simulink model "LUTtest"  (R2021b)
settings: Solver=FixedStepAuto  StartTime=0.0  StopTime=20  RelTol=1e-3  EnableMultiTasking=on
model workspace (MAT data in the model file):
  lutSpeed = Simulink.LookupTable
  lutSpeed.Table = Simulink.lookuptable.Table
  lutSpeed.Table.Value = [-0.999909204263 -0.999329299739 -0.995054753687 -0.964027580076 -0.761594155956 0 0.761594155956 0.964027580076 0.995054753687 0.999329299739 0.999909204263]
  lutSpeed.Table.Dimensions = [1 11]
  lutSpeed.Table.DataType = 'auto'
  lutSpeed.Table.FieldName = 'Table'
  lutSpeed.Breakpoints = Simulink.lookuptable.Breakpoint
  lutSpeed.Breakpoints.Value = [-5 -4 -3 -2 -1 0 1 2 3 4 5]
  lutSpeed.Breakpoints.TunableSizeName = 'N1'
  lutSpeed.Breakpoints.Dimensions = [1 11]
  lutSpeed.Breakpoints.DataType = 'auto'
  lutSpeed.Breakpoints.FieldName = 'BP1'
  lutSpeed.SupportTunableSize = 0
  lutSpeed.StructTypeInfo = Simulink.lookuptable.StructTypeInfo
  lutSpeed.StructTypeInfo.Name = 'lutSpeed'
  lutSpeed.StructTypeInfo.DataScope = 'Auto'
  pwm_speed = Simulink.LookupTable
  pwm_speed.Table = Simulink.lookuptable.Table
  pwm_speed.Table.Value = [-0.999909204263 -0.999329299739 -0.995054753687 -0.964027580076 -0.761594155956 0 0.761594155956 0.964027580076 0.995054753687 0.999329299739 0.999909204263]
  pwm_speed.Table.Dimensions = [1 11]
  pwm_speed.Table.DataType = 'auto'
  pwm_speed.Table.FieldName = 'Table'
  pwm_speed.Breakpoints = Simulink.lookuptable.Breakpoint
  pwm_speed.Breakpoints.Value = [-5 -4 -3 -2 -1 0 1 2 3 4 5]
  pwm_speed.Breakpoints.TunableSizeName = 'N1'
  pwm_speed.Breakpoints.Dimensions = [1 11]
  pwm_speed.Breakpoints.DataType = 'auto'
  pwm_speed.Breakpoints.FieldName = 'BP1'
  pwm_speed.SupportTunableSize = 0
  pwm_speed.StructTypeInfo = Simulink.lookuptable.StructTypeInfo
  pwm_speed.StructTypeInfo.Name = 'pwm_speed'
  pwm_speed.StructTypeInfo.DataScope = 'Auto'
undefined symbols (not defined in the file or in its folder): sigbuilder_block
settings Model: ExtModeTrigDuration=2  Creator=yo  LastModifiedBy=yo
settings OptimizationCC: EnhancedBackFolding=on  PassReuseOutputArgsAs=Individual arguments  ZeroExternalMemoryAtStartup=off  ZeroInternalMemoryAtStartup=off  MaxStackSize=64  OptimizeBlockOrder=speed  DifferentSizesBufferReuse=on  OptimizationCustomize=off  EfficientTunableParamExpr=on
settings DebuggingCC: ParameterTunabilityLossMsg=error
settings HardwareCC: ProdBitPerInt=16  ProdBitPerPointer=16  ProdBitPerSizeT=16  ProdBitPerPtrDiffT=16  ProdLargestAtomicFloat=None  ProdWordSize=8  ProdHWDeviceType=Atmel->AVR  UseEmbeddedCoderFeatures=off  UseSimulinkCoderFeatures=off
settings SFSimCC: MATLABDynamicMemAlloc=off
settings RTWCC: Description=Embedded Coder  SystemTargetFile=ert.tlc  HardwareBoard=Arduino Mega 2560  TemplateMakefile=ert_default_tmf  Toolchain=Arduino AVR  BuildConfiguration=Faster Runs
settings CodeAppCC: ForceParamTrailComments=on  IgnoreCustomStorageClasses=off  OperatorAnnotations=on  SimulinkDataObjDesc=on  SFDataObjDesc=on  InsertBlockDesc=on
settings ERTTargetCC: SupportContinuousTime=on  SupportNonInlinedSFcns=on  SupportVariableSizeSignals=on  ExtModeTransport=3  ExtModeStaticAlloc=on  ExtModeStaticAllocSize=2048  ExtModeMexFile=ext_xcp  ExtModeIntrfLevel=Level2 - Open

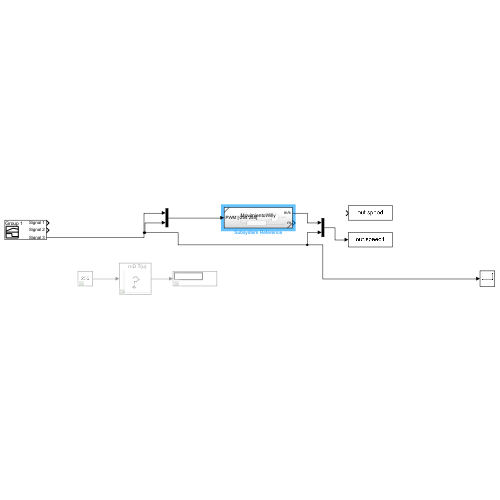
[thumbnail: Simulink's stored preview of the top-level diagram]
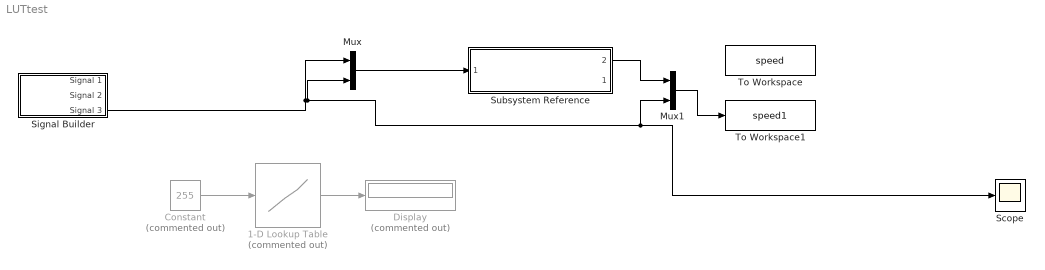
== system LUTtest ==
  1-D Lookup Table : Lookup_n-D  Commented=on  NumberOfTableDimensions=1  BreakpointsForDimension1=[0.614242553710938,0.535507202148438,0.440994262695313,0.31500244140625,0.188995361328125,0.078765869140625,0,-0.1732177734375,-0.28350830078125,-0.42529296875,-0.535491943359375,-0.645736694335938]  Table=[255,209.099990844727,163.200012207031,117.300010681152,71.4000244140625,25.5,-21.4199905395508,-67.3199768066406,-113.219970703125,-159.119995117188,-205.019989013672,-255]  InternalRulePriority=Speed  RndMeth=Simplest  InputSameDT=on
  Constant : Constant  Commented=on  Value=255
  Display : Display  Commented=on
  Mux : Mux  Inputs=2
  Mux1 : Mux  Inputs=2
  Scope : Scope
  Signal Builder : Subsystem  Tag=STV Subsys  LoadFcn=sigbuilder_block('load');  StartFcn=sigbuilder_block('start');  StopFcn=sigbuilder_block('stop');  ClipboardFcn=sigbuilder_block('clipboard');  mask(Sigbuilder block){tuvar=[0:10]}
      mask help: Simulink:masks:SigbuilderBlock_MD
      mask init:
      | if ~strcmp(get_param(bdroot(gcbh),'SimulationStatus'),'stopped') tuvar = sigbuilder_block('maskInit'); end
      settings: CopyFcn=sigbuilder_block('copy');  DeleteFcn=sigbuilder_block('delete');  ModelCloseFcn=sigbuilder_block('modelClose');  PreSaveFcn=sigbuilder_block('preSave');  PauseFcn=sigbuilder_block('pause');  ContinueFcn=sigbuilder_block('continue');  NameChangeFcn=sigbuilder_block('namechange');  OpenFcn=sigbuilder_block('open',[5.4 0 1141.2 552.6 ]);  CloseFcn=sigbuilder_block('close');
      mask Display: plot(0, 0, 100, 100,[2, 2, 32, 32, 2], [68, 8, 8, 68, 68],[32, 2], [38, 38], [32, 19, 2],[53, 60, 44], [32, 17, 17, 2],[16, 16, 31, 31]);txt = getActiveGroup(gcbh);text(2, 100, txt,'verticalAlignment', 'top');
  Subsystem Reference : Subsystem  ReferencedSubsystem=MovimientoWilly
      settings: PortSchema="{\"entries\":[{\"content\":{\"sides\":[{\"content\":{\"connectorIds\":[\"In1\"]},\"type\":\"ConnectorPlacement.EquallySpacedRectSide\",\"uuid\":\"e2e62d12-b901-4b36-ba0a-f7966db22eb1\"},{\"content\":{\"connectorIds\":[\"Out2\",\"Out1\"],\"side\":\"RIGHT\"},\"type\":\"ConnectorPlacement.EquallySpacedRectSide\",\"uuid\":\"4ac40844-dd86-4583-85d0-1a3dbcadadf6\"},{\"content\":{\"connectorIds\":[],\"side\":\"TOP\"},\"type\":\"ConnectorPlacement.EquallySpacedRectSide\",\"uuid\":\"ba3c34be-1fcf-4864-8518-3c5c018d879c\"}]},\"type\":\"ConnectorPlacement.EquallySpacedConnector\",\"uuid\":\"5341ca39-b1d9-450b-91b0-88ff8703ff82\"}],\"packageUris\":[\"http://schema.mathworks.com/mf0/Connector/R2020b\"],\"version\":\"1.0\"}"
  To Workspace : ToWorkspace  VariableName=speed  SampleTime=-1
      settings: Save2DSignal=2-D array (concatenate along first dimension)
  To Workspace1 : ToWorkspace  VariableName=speed1  SampleTime=-1
      settings: Save2DSignal=2-D array (concatenate along first dimension)
  wires:
  Subsystem Reference/2 -> Mux1/1
  Mux/1 -> Subsystem Reference/1
  Signal Builder/3(Signal 3) -> Mux/1, Mux/2, Mux1/2, Scope/1
  Mux1/1 -> To Workspace1/1
  1-D Lookup Table/1 -> Display/1
  Constant/1 -> 1-D Lookup Table/1

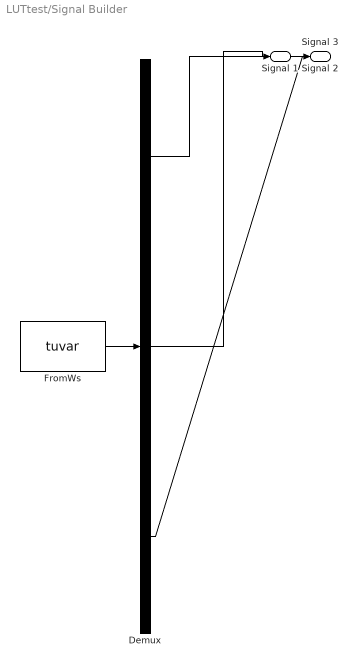
== system LUTtest/Signal Builder ==
  Demux : Demux  Tag=STV Demux  Outputs=3
      settings: DisplayOption=none
  FromWs : FromWorkspace  Tag=STV FromWs  VariableName=tuvar
      SigBuilderData=|
      | common.afterFinalStr = 'Extrapolate'
      | common.sampleTime = 0
      | dataSet.timeRange = [0 15]
      | dataSet.name = 'Group 1'
      | sbobj.Groups.Name = 'Group 1'
      | sbobj.Groups.Signals(1).Name = 'Signal 1'
      | sbobj.Groups.Signals(1).XData = [0 4 4 6 6 15]
      | sbobj.Groups.Signals(1).YData = [0 0 1 1 0 0]
      | sbobj.Groups.Signals(2).Name = 'Signal 2'
      | sbobj.Groups.Signals(2).XData = [0 2 4 4 8 8 10 15]
      | sbobj.Groups.Signals(2).YData = [0 0 254.9 -255.1 254.9 -255.1 0 0]
      | sbobj.Groups.Signals(3).Name = 'Signal 3'
      | sbobj.Groups.Signals(3).XData = [0 2 4 8 8 15]
      | sbobj.Groups.Signals(3).YData = [0 0 255 -255 0 0]
      | sbobj.Groups.TimeRange = [0 15]
  Signal 1 : Outport  Tag=STV Outport
  Signal 2 : Outport  Tag=STV Outport  Port=2
  Signal 3 : Outport  Tag=STV Outport  Port=3
  wires:
  Demux/1 -> Signal 1/1
  FromWs/1 -> Demux/1
  Demux/2 -> Signal 2/1
  Demux/3 -> Signal 3/1
